simulink model "LAB4_Euler_eq_Euler_angles"  (R2022b)
settings: Solver=ode4  StartTime=0.0  StopTime=100  FixedStep=0.1  RelTol=1e-3
values from neighbouring files (symbols this model uses):
  euler_angles_0 = [1;1;1]    [LAB_03.m]
  I = diag([0.025 , 0.055 , 0.07])    [LAB_03.m]
  w0 = [2*pi , 1 , 0.1]    [LAB_03.m]
libraries: sharedutil x3, matrix_library x1
settings Model: Creator=ludov  LastModifiedBy=ludov

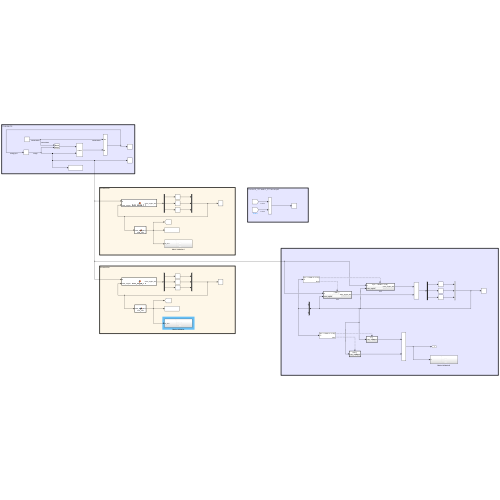
[thumbnail: Simulink's stored preview of the top-level diagram]
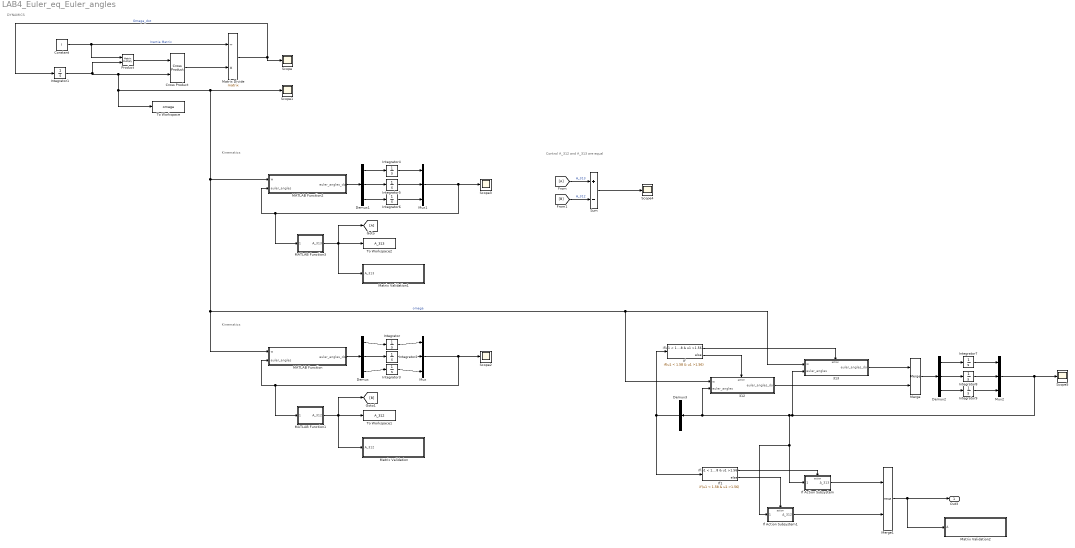
== system LAB4_Euler_eq_Euler_angles ==
  note: Control A_312 and A_313 are equal
  note: Kinematics
  note: DYNAMICS
  note: Kinematics
  312 : Subsystem  TreatAsAtomicUnit=on
  313 : Subsystem  TreatAsAtomicUnit=on
  Constant : Constant  Value=I
  Cross Product : matrix_library/Cross Product
  Demux{,1..3} (4 alike) : Demux  Outputs=3
  From : From
  Goto : Goto
  If : If  IfExpression=u1 < 1.58 & u1 >1.56
  If Action Subsystem : Subsystem  TreatAsAtomicUnit=on
  If Action Subsystem1 : Subsystem  TreatAsAtomicUnit=on
  If1 : If  IfExpression=u1 < 1.58 & u1 >1.56
  Integrator : Integrator  InitialCondition=euler_angles_0(1)  WrapState=on  WrappedStateUpperValue=2*pi  WrappedStateLowerValue=0
  Integrator1 : Integrator  InitialCondition=w0
  Integrator2 : Integrator  InitialCondition=euler_angles_0(2)  WrapState=on
  Integrator3 : Integrator  InitialCondition=euler_angles_0(3)  WrapState=on  WrappedStateUpperValue=2*pi  WrappedStateLowerValue=0
  Integrator4 : Integrator  InitialCondition=euler_angles_0(1)  WrapState=on  WrappedStateUpperValue=2*pi  WrappedStateLowerValue=0
  Integrator5 : Integrator  InitialCondition=euler_angles_0(2)  WrapState=on
  Integrator6 : Integrator  InitialCondition=euler_angles_0(3)  WrapState=on  WrappedStateUpperValue=2*pi  WrappedStateLowerValue=0
  Integrator7 : Integrator  InitialCondition=euler_angles_0(1)  WrapState=on  WrappedStateUpperValue=2*pi  WrappedStateLowerValue=0
  Integrator8 : Integrator  InitialCondition=euler_angles_0(2)  WrapState=on
  Integrator9 : Integrator  InitialCondition=euler_angles_0(3)  WrapState=on  WrappedStateUpperValue=2*pi  WrappedStateLowerValue=0
  MATLAB Function : MATLAB Function  TreatAsAtomicUnit=on
  MATLAB Function1 : MATLAB Function  TreatAsAtomicUnit=on
  MATLAB Function2 : MATLAB Function  TreatAsAtomicUnit=on
  MATLAB Function3 : MATLAB Function  TreatAsAtomicUnit=on
  Matrix Divide : Product  Inputs=/*  Multiplication=Matrix(*)
  Matrix Validation : Subsystem
  Matrix Validation1 : Subsystem
  Matrix Validation2 : Subsystem
  Merge : Merge
  Merge1 : Merge
  Mux : Mux  Inputs=3
  Mux1 : Mux  Inputs=3
  Mux2 : Mux  Inputs=3
  Product : Product  Multiplication=Matrix(*)
  Scope{,1..5} (6 alike) : Scope
  Sum : Sum  Inputs=+-
  To Workspace : ToWorkspace  VariableName=omega  SaveFormat=Timeseries  SampleTime=-1
  To Workspace1 : ToWorkspace  VariableName=A_312  SaveFormat=Timeseries  SampleTime=-1
  To Workspace2 : ToWorkspace  VariableName=A_313  SaveFormat=Timeseries  SampleTime=-1
  Out3 : Outport
  wires:
  Constant/1 -> Product/1, Matrix Divide/1  "Inertia Matrix"
  Product/1 -> Cross Product/1
  Cross Product/1 -> Matrix Divide/2
  Matrix Divide/1 -> Integrator1/1, Scope/1  "Omega_dot"
  MATLAB Function/1(euler_angles_dot) -> Demux/1
  MATLAB Function1/1(A_312) -> [B], Matrix Validation/1(A_312), To Workspace1/1
  Demux/1 -> Integrator/1
  Integrator/1 -> Mux/1
  Demux/2 -> Integrator2/1
  Integrator2/1 -> Mux/2
  Demux/3 -> Integrator3/1
  Integrator3/1 -> Mux/3
  Mux/1 -> Scope2/1, MATLAB Function1/1(euler_angles), MATLAB Function/2(euler_angles)
  Demux1/3 -> Integrator6/1
  MATLAB Function2/1(euler_angles_dot) -> Demux1/1
  Demux1/2 -> Integrator5/1
  Integrator5/1 -> Mux1/2
  MATLAB Function3/1(A_313) -> Goto/1, Matrix Validation1/1(A_313), To Workspace2/1
  Demux1/1 -> Integrator4/1
  Integrator4/1 -> Mux1/1
  Integrator6/1 -> Mux1/3
  Mux1/1 -> Scope3/1, MATLAB Function3/1(euler_angles), MATLAB Function2/2(euler_angles)
  From/1 -> Sum/1  "A_313"
  [B] -> Sum/2  "A_312"
  Sum/1 -> Scope4/1
  Integrator1/1 -> To Workspace/1, MATLAB Function2/1(w), MATLAB Function/1(w), 312/1(w), 313/1(w), Scope1/1, Cross Product/2, Product/2  "omega"
  If/1 -> 313/Action
  If/2 -> 312/Action
  Mux2/1 -> Scope5/1, 313/2(euler_angles), 312/2(euler_angles), Demux3/1, If Action Subsystem1/1(euler_angles), If Action Subsystem/1(euler_angles)
  313/1(euler_angles_dot) -> Merge/1
  312/1(euler_angles_dot) -> Merge/2
  Demux2/3 -> Integrator9/1
  Merge/1 -> Demux2/1
  Demux2/2 -> Integrator8/1
  Integrator7/1 -> Mux2/1
  Demux2/1 -> Integrator7/1
  Integrator8/1 -> Mux2/2
  Integrator9/1 -> Mux2/3
  Demux3/2 -> If1/1, If/1
  If1/1 -> If Action Subsystem/Action
  If1/2 -> If Action Subsystem1/Action
  If Action Subsystem/1(A_313) -> Merge1/1
  If Action Subsystem1/1(A_312) -> Merge1/2
  Merge1/1 -> Matrix Validation2/1(A), Out3/1

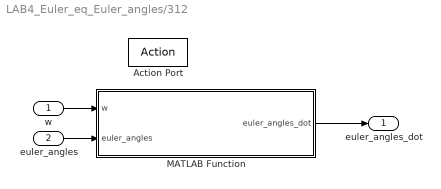
== system LAB4_Euler_eq_Euler_angles/312 ==
  w : Inport
  euler_angles : Inport  Port=2
  Action Port : ActionPort  ActionPortLabel=else
  MATLAB Function : MATLAB Function  TreatAsAtomicUnit=on
  euler_angles_dot : Outport
  wires:
  w/1 -> MATLAB Function/1(w)
  euler_angles/1 -> MATLAB Function/2(euler_angles)
  MATLAB Function/1(euler_angles_dot) -> euler_angles_dot/1

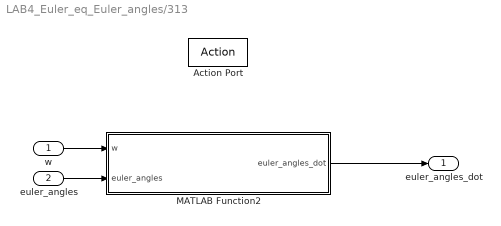
== system LAB4_Euler_eq_Euler_angles/313 ==
  w : Inport
  euler_angles : Inport  Port=2
  Action Port : ActionPort  ActionPortLabel=if(u1 < 1.58 & u1 >1.56)
  MATLAB Function2 : MATLAB Function  TreatAsAtomicUnit=on
  euler_angles_dot : Outport
  wires:
  w/1 -> MATLAB Function2/1(w)
  euler_angles/1 -> MATLAB Function2/2(euler_angles)
  MATLAB Function2/1(euler_angles_dot) -> euler_angles_dot/1

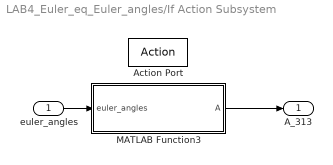
== system LAB4_Euler_eq_Euler_angles/If Action Subsystem ==
  euler_angles : Inport
  Action Port : ActionPort  ActionPortLabel=if(u1 < 1.58 & u1 >1.56)
  MATLAB Function3 : MATLAB Function  TreatAsAtomicUnit=on
  A_313 : Outport
  wires:
  euler_angles/1 -> MATLAB Function3/1(euler_angles)
  MATLAB Function3/1(A) -> A_313/1

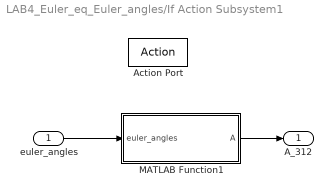
== system LAB4_Euler_eq_Euler_angles/If Action Subsystem1 ==
  euler_angles : Inport
  Action Port : ActionPort  ActionPortLabel=else
  MATLAB Function1 : MATLAB Function  TreatAsAtomicUnit=on
  A_312 : Outport
  wires:
  euler_angles/1 -> MATLAB Function1/1(euler_angles)
  MATLAB Function1/1(A) -> A_312/1

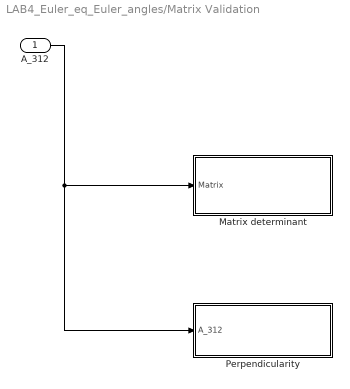
== system LAB4_Euler_eq_Euler_angles/Matrix Validation ==
  A_312 : Inport
  Matrix determinant : Subsystem
  Perpendicularity : Subsystem
  wires:
  A_312/1 -> Perpendicularity/1(A_312), Matrix determinant/1(Matrix)

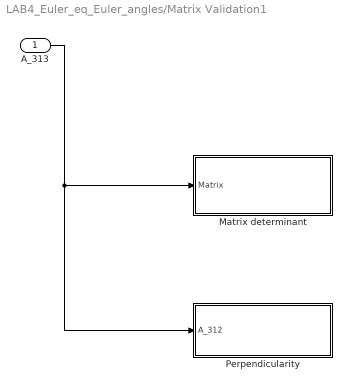
== system LAB4_Euler_eq_Euler_angles/Matrix Validation1 ==
  A_313 : Inport
  Matrix determinant : Subsystem
  Perpendicularity : Subsystem
  wires:
  A_313/1 -> Perpendicularity/1(A_312), Matrix determinant/1(Matrix)

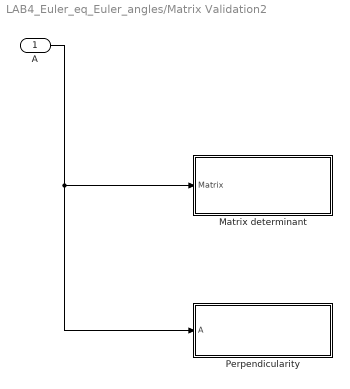
== system LAB4_Euler_eq_Euler_angles/Matrix Validation2 ==
  A : Inport
  Matrix determinant : Subsystem
  Perpendicularity : Subsystem
  wires:
  A/1 -> Perpendicularity/1(A), Matrix determinant/1(Matrix)

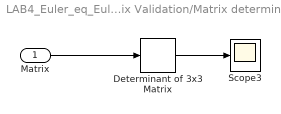
== system LAB4_Euler_eq_Euler_angles/Matrix Validation/Matrix determinant ==
  Matrix : Inport
  Determinant of 3x3 Matrix : sharedutil/Determinant of 3x3 Matrix  aMode=aMode
      settings: LibrarySourceBlock=|
      | aerolibutil/Determinant of
      | 3x3 Matrix
  Scope3 : Scope
  wires:
  Determinant of 3x3 Matrix/1 -> Scope3/1
  Matrix/1 -> Determinant of 3x3 Matrix/1

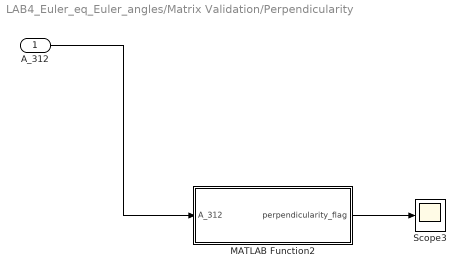
== system LAB4_Euler_eq_Euler_angles/Matrix Validation/Perpendicularity ==
  A_312 : Inport
  MATLAB Function2 : MATLAB Function  TreatAsAtomicUnit=on
  Scope3 : Scope
  wires:
  MATLAB Function2/1(perpendicularity_flag) -> Scope3/1
  A_312/1 -> MATLAB Function2/1(A_312)

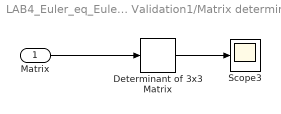
== system LAB4_Euler_eq_Euler_angles/Matrix Validation1/Matrix determinant ==
  Matrix : Inport
  Determinant of 3x3 Matrix : sharedutil/Determinant of 3x3 Matrix  aMode=aMode
      settings: LibrarySourceBlock=|
      | aerolibutil/Determinant of
      | 3x3 Matrix
  Scope3 : Scope
  wires:
  Determinant of 3x3 Matrix/1 -> Scope3/1
  Matrix/1 -> Determinant of 3x3 Matrix/1

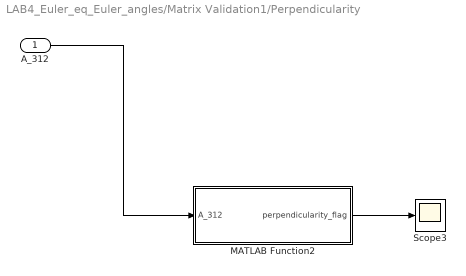
== system LAB4_Euler_eq_Euler_angles/Matrix Validation1/Perpendicularity ==
  A_312 : Inport
  MATLAB Function2 : MATLAB Function  TreatAsAtomicUnit=on
  Scope3 : Scope
  wires:
  MATLAB Function2/1(perpendicularity_flag) -> Scope3/1
  A_312/1 -> MATLAB Function2/1(A_312)

== system LAB4_Euler_eq_Euler_angles/Matrix Validation2/Matrix determinant ==
  Matrix : Inport
  Determinant of 3x3 Matrix : sharedutil/Determinant of 3x3 Matrix  aMode=aMode
      settings: LibrarySourceBlock=|
      | aerolibutil/Determinant of
      | 3x3 Matrix
  Scope3 : Scope
  wires:
  Determinant of 3x3 Matrix/1 -> Scope3/1
  Matrix/1 -> Determinant of 3x3 Matrix/1

== system LAB4_Euler_eq_Euler_angles/Matrix Validation2/Perpendicularity ==
  A : Inport
  MATLAB Function2 : MATLAB Function  TreatAsAtomicUnit=on
  Scope3 : Scope
  wires:
  MATLAB Function2/1(perpendicularity_flag) -> Scope3/1
  A/1 -> MATLAB Function2/1(A)

== matlab function LAB4_Euler_eq_Euler_angles/MATLAB Function1 ==
  data: euler_angles input; A_312 output
function A_312 = DCM_312(euler_angles)

% Define data
    phi         = euler_angles(1);
    theta       = euler_angles(2);
    psi         = euler_angles(3);

A_312=[ cos(psi)*cos(phi) - sin(psi)*sin(phi)*sin(theta)     , cos(psi)*sin(phi) + sin(psi)*cos(phi)*sin(theta)  , -sin(psi)*cos(theta)  ;
        -sin(phi)*cos(theta)                                 , cos(phi)*cos(theta)                               , sin(theta)            ;
        sin(psi)*cos(phi) + cos(psi)*sin(phi)*sin(theta)     , sin(psi)*sin(phi) - cos(psi)*cos(phi)*sin(theta)  , cos(theta)*cos(psi)   ];
end

== matlab function LAB4_Euler_eq_Euler_angles/MATLAB Function ==
  data: w input; euler_angles_dot output; euler_angles input
function euler_angles_dot = Euler_angles_312(w, euler_angles)
    
% Define data
    phi         = euler_angles(1);
    theta       = euler_angles(2);
    psi         = euler_angles(3);

% Calculate derivatives of Euler's angles 312
     phi_dot     = (w(3)*cos(psi) - w(1)*sin(psi))/cos(theta);
     theta_dot   = w(1)*cos(psi) + w(3)*sin(psi);
     psi_dot     = w(2) - (w(3)*cos(psi) - w(1)*sin(psi)) * (sin(theta)/cos(theta));


    
% Calculate derivatives of Euler's angles 313
%     phi_dot     = (w(1)*sin(psi) + w(2)*cos(psi))/sin(theta);
%     theta_dot   = w(1)*cos(psi) - w(2)*sin(psi);
%     psi_dot     = w(3) - (w(1)*sin(psi) + w(2)*cos(psi)) * (cos(theta)/sin(theta));

    euler_angles_dot=[phi_dot;theta_dot;psi_dot];


end

== matlab function LAB4_Euler_eq_Euler_angles/Matrix Validation/Perpendicularity/MATLAB Function2 ==
  data: A_312 input; perpendicularity_flag output
function perpendicularity_flag = fcn(A_312)
    

perpendicularity_flag =zeros(3,1);

    x   = A_312(1,:);
    y   = A_312(2,:);
    z   = A_312(3,:);

    perpendicularity_flag(1)=dot(x,y);
    perpendicularity_flag(2)=dot(x,z);
    perpendicularity_flag(1)=dot(z,y);

end

== matlab function LAB4_Euler_eq_Euler_angles/MATLAB Function2 ==
  data: w input; euler_angles_dot output; euler_angles input
function euler_angles_dot = Euler_angles_313(w, euler_angles)
    
% Define data
    phi         = euler_angles(1);
    theta       = euler_angles(2);
    psi         = euler_angles(3);

    
% Calculate derivatives of Euler's angles 313
     phi_dot     = (w(1)*sin(psi) + w(2)*cos(psi))/sin(theta);
     theta_dot   = w(1)*cos(psi) - w(2)*sin(psi);
     psi_dot     = w(3) - (w(1)*sin(psi) + w(2)*cos(psi)) * (cos(theta)/sin(theta));

    euler_angles_dot=[phi_dot;theta_dot;psi_dot];


end

== matlab function LAB4_Euler_eq_Euler_angles/MATLAB Function3 ==
  data: euler_angles input; A_313 output
function A_313 = DCM_313(euler_angles)

% Define data
    phi         = euler_angles(1);
    theta       = euler_angles(2);
    psi         = euler_angles(3);

A_313=[ cos(psi)*cos(phi) - sin(psi)*sin(phi)*cos(theta)     , cos(psi)*sin(phi) + sin(psi)*cos(phi)*cos(theta)     , sin(psi)*sin(theta)  ;
        - sin(psi)*cos(phi) - cos(psi)*sin(phi)*cos(theta)   , - sin(psi)*sin(phi) + cos(psi)*cos(phi)*cos(theta)   , sin(theta)*cos(psi)  ;
        sin(phi)*sin(theta)                                  , - cos(phi)*sin(theta)                                , cos(theta)           ];
end

== matlab function LAB4_Euler_eq_Euler_angles/Matrix Validation1/Perpendicularity/MATLAB Function2 ==
  data: A_312 input; perpendicularity_flag output
function perpendicularity_flag = fcn(A_312)
    

perpendicularity_flag =zeros(3,1);

    x   = A_312(1,:);
    y   = A_312(2,:);
    z   = A_312(3,:);

    perpendicularity_flag(1)=dot(x,y);
    perpendicularity_flag(2)=dot(x,z);
    perpendicularity_flag(1)=dot(z,y);

end

== matlab function LAB4_Euler_eq_Euler_angles/313/MATLAB Function2 ==
  data: w input; euler_angles_dot output; euler_angles input
function euler_angles_dot = Euler_angles_313(w, euler_angles)
    
% Define data
    phi         = euler_angles(1);
    theta       = euler_angles(2);
    psi         = euler_angles(3);

    
% Calculate derivatives of Euler's angles 313
     phi_dot     = (w(1)*sin(psi) + w(2)*cos(psi))/sin(theta);
     theta_dot   = w(1)*cos(psi) - w(2)*sin(psi);
     psi_dot     = w(3) - (w(1)*sin(psi) + w(2)*cos(psi)) * (cos(theta)/sin(theta));

    euler_angles_dot=[phi_dot;theta_dot;psi_dot];


end

== matlab function LAB4_Euler_eq_Euler_angles/312/MATLAB Function ==
  data: w input; euler_angles_dot output; euler_angles input
function euler_angles_dot = Euler_angles_312(w, euler_angles)
    
% Define data
    phi         = euler_angles(1);
    theta       = euler_angles(2);
    psi         = euler_angles(3);

% Calculate derivatives of Euler's angles 312
     phi_dot     = (w(3)*cos(psi) - w(1)*sin(psi))/cos(theta);
     theta_dot   = w(1)*cos(psi) + w(3)*sin(psi);
     psi_dot     = w(2) - (w(3)*cos(psi) - w(1)*sin(psi)) * (sin(theta)/cos(theta));


    
% Calculate derivatives of Euler's angles 313
%     phi_dot     = (w(1)*sin(psi) + w(2)*cos(psi))/sin(theta);
%     theta_dot   = w(1)*cos(psi) - w(2)*sin(psi);
%     psi_dot     = w(3) - (w(1)*sin(psi) + w(2)*cos(psi)) * (cos(theta)/sin(theta));

    euler_angles_dot=[phi_dot;theta_dot;psi_dot];


end

== matlab function LAB4_Euler_eq_Euler_angles/If Action Subsystem/MATLAB Function3 ==
  data: euler_angles input; A output
function A = DCM_313(euler_angles)

% Define data
    phi         = euler_angles(1);
    theta       = euler_angles(2);
    psi         = euler_angles(3);

A=[ cos(psi)*cos(phi) + sin(psi)*sin(phi)*cos(theta)     , cos(psi)*sin(phi) + sin(psi)*cos(phi)*cos(theta)     , sin(psi)*sin(theta)  ;
        - sin(psi)*cos(phi) - cos(psi)*sin(phi)*cos(theta)   , - sin(psi)*sin(phi) + cos(psi)*cos(phi)*cos(theta)   , sin(theta)*cos(psi)  ;
        sin(phi)*sin(theta)                                  , - cos(phi)*sin(theta)                                  , cos(theta)         ];
end

== matlab function LAB4_Euler_eq_Euler_angles/If Action Subsystem1/MATLAB Function1 ==
  data: euler_angles input; A output
function A = DCM_312(euler_angles)

% Define data
    phi         = euler_angles(1);
    theta       = euler_angles(2);
    psi         = euler_angles(3);

A=[ cos(psi)*cos(phi) - sin(psi)*sin(phi)*sin(theta)     , cos(psi)*sin(phi) + sin(psi)*cos(phi)*sin(theta)  , -sin(psi)*cos(theta)  ;
        -sin(phi)*cos(theta)                                 , cos(phi)*cos(theta)                               , sin(theta)            ;
        sin(psi)*cos(phi) + cos(psi)*sin(phi)*sin(theta)     , sin(psi)*sin(phi) - cos(psi)*cos(phi)*sin(theta)  , cos(theta)*cos(psi)   ];
end

== matlab function LAB4_Euler_eq_Euler_angles/Matrix Validation2/Perpendicularity/MATLAB Function2 ==
  data: A input; perpendicularity_flag output
function perpendicularity_flag = fcn(A)
    

perpendicularity_flag =zeros(3,1);

    x   = A(1,:);
    y   = A(2,:);
    z   = A(3,:);

    perpendicularity_flag(1)=dot(x,y);
    perpendicularity_flag(2)=dot(x,z);
    perpendicularity_flag(1)=dot(z,y);

end
